simulink model "Oppg2"  (R2021b)
settings: Solver=VariableStepAuto  StartTime=0.0  StopTime=100  RelTol=1e-3
settings Model: Creator=rezoan  LastModifiedBy=rezoan

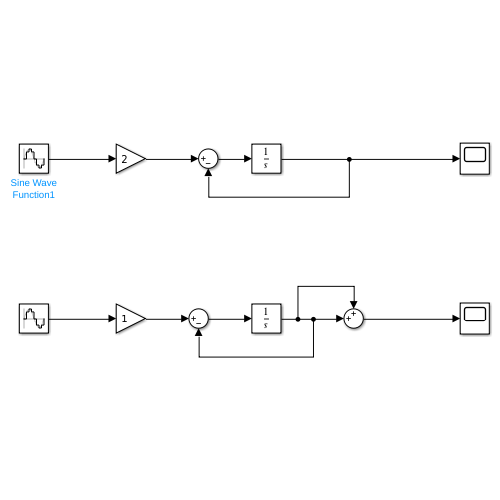
[thumbnail: Simulink's stored preview of the top-level diagram]
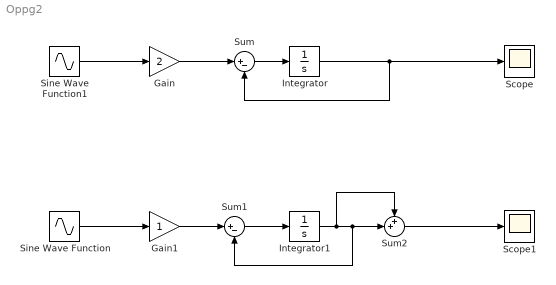
== system Oppg2 ==
  Gain : Gain  Gain=2
  Gain1 : Gain
  Integrator : Integrator
  Integrator1 : Integrator
  Scope : Scope
  Scope1 : Scope
  Sine Wave Function : Sin  Frequency=10  SampleTime=0.1
  Sine Wave Function1 : Sin  Frequency=100  SampleTime=0.01
  Sum : Sum  Inputs=|+-
  Sum1 : Sum  Inputs=|+-
  Sum2 : Sum  Inputs=++|
  wires:
  Gain/1 -> Sum/1
  Sum/1 -> Integrator/1
  Integrator/1 -> Scope/1, Sum/2
  Sine Wave Function/1 -> Gain1/1
  Gain1/1 -> Sum1/1
  Sum1/1 -> Integrator1/1
  Sum2/1 -> Scope1/1
  Integrator1/1 -> Sum2/1, Sum1/2, Sum2/2
  Sine Wave Function1/1 -> Gain/1
